simulink model "maze_solver"  (R2026a)
settings: Solver=FixedStepDiscrete  StopTime=1  FixedStep=0.01
InitFcn:
  | run(fullfile(currentProject().RootFolder,'config','robot_params.m'))
undefined symbols (not defined in the file): DiscIntNeverNeededParam, motor, robot, Ts
settings Model: Creator=richs  LastModifiedBy=richs

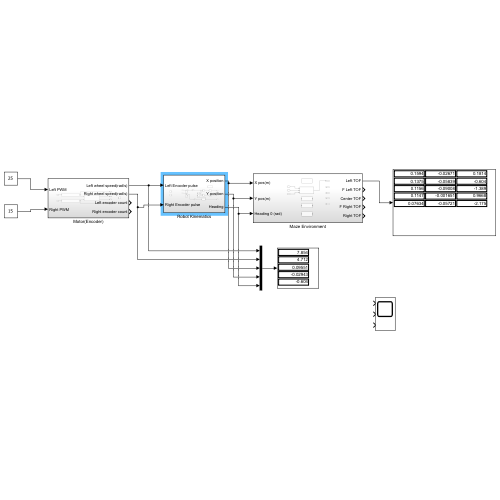
[thumbnail: Simulink's stored preview of the top-level diagram]
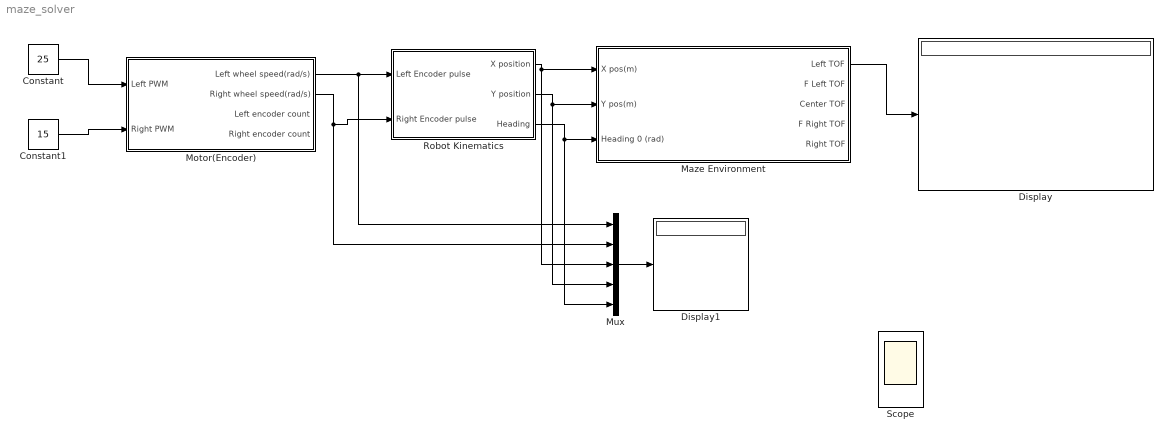
== system maze_solver ==
  Constant : Constant  Value=25
  Constant1 : Constant  Value=15
  Display : Display
  Display1 : Display
  Maze Environment : Subsystem
  Motor(Encoder) : Subsystem
  Mux : Mux  Inputs=5
  Robot Kinematics : Subsystem
  Scope : Scope  NumInputPorts=3
      settings: ActiveDisplayYMinimum=-0.29962469310207057  ActiveDisplayYMaximum=0.042415818455105447
  wires:
  Motor(Encoder)/1(Left wheel speed(rad/s)) -> Mux/1, Robot Kinematics/1(Left Encoder pulse)
  Motor(Encoder)/2(Right wheel speed(rad/s)) -> Mux/2, Robot Kinematics/2(Right Encoder pulse)
  Constant/1 -> Motor(Encoder)/1(Left PWM)
  Constant1/1 -> Motor(Encoder)/2(Right PWM)
  Robot Kinematics/1(X position) -> Mux/3, Maze Environment/1(X pos(m))
  Robot Kinematics/2(Y position) -> Mux/4, Maze Environment/2(Y pos(m))
  Robot Kinematics/3(Heading) -> Mux/5, Maze Environment/3(Heading 0 (rad))
  Mux/1 -> Display1/1
  Maze Environment/1(Left TOF) -> Display/1

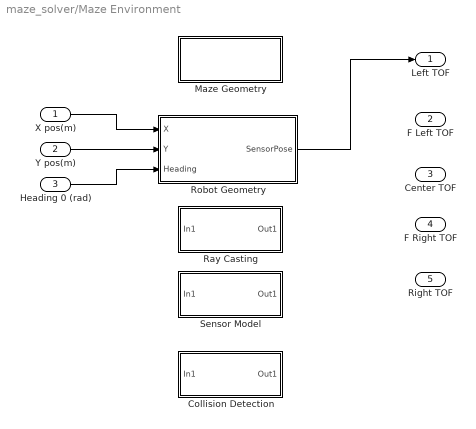
== system maze_solver/Maze Environment ==
  X pos(m) : Inport
  Y pos(m) : Inport  Port=2
  Heading 0 (rad) : Inport  Port=3
  Collision Detection : Subsystem
  Maze Geometry : Subsystem
  Ray Casting : Subsystem
  Robot Geometry : Subsystem
  Sensor Model : Subsystem
  Left TOF : Outport
  F Left TOF : Outport  Port=2
  Center TOF : Outport  Port=3
  F Right TOF : Outport  Port=4
  Right TOF : Outport  Port=5
  wires:
  X pos(m)/1 -> Robot Geometry/1(X)
  Y pos(m)/1 -> Robot Geometry/2(Y)
  Heading 0 (rad)/1 -> Robot Geometry/3(Heading)
  Robot Geometry/1(SensorPose) -> Left TOF/1

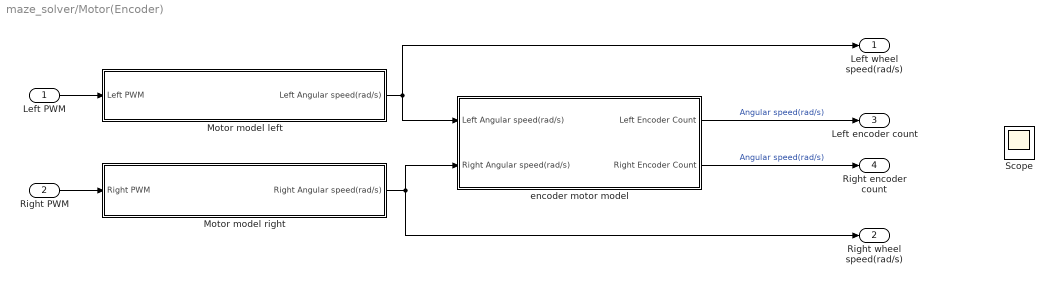
== system maze_solver/Motor(Encoder) ==
  Left PWM : Inport
  Right PWM : Inport  Port=2
  Motor model left : Subsystem
  Motor model right : Subsystem
  Scope : Scope  NumInputPorts=2
      settings: ActiveDisplayYMinimum=259.90483016263516  ActiveDisplayYMaximum=297.8633074912612
  encoder motor model : Subsystem
  Left wheel speed(rad/s) : Outport
  Right wheel speed(rad/s) : Outport  Port=2
  Left encoder count : Outport  Port=3
  Right encoder count : Outport  Port=4
  wires:
  Motor model left/1(Left Angular speed(rad/s)) -> encoder motor model/1(Left Angular speed(rad/s)), Left wheel speed(rad/s)/1
  Motor model right/1(Right Angular speed(rad/s)) -> Right wheel speed(rad/s)/1, encoder motor model/2(Right Angular speed(rad/s))
  Left PWM/1 -> Motor model left/1(Left PWM)
  Right PWM/1 -> Motor model right/1(Right PWM)
  encoder motor model/1(Left Encoder Count) -> Left encoder count/1  "Angular speed(rad/s)"
  encoder motor model/2(Right Encoder Count) -> Right encoder count/1  "Angular speed(rad/s)"

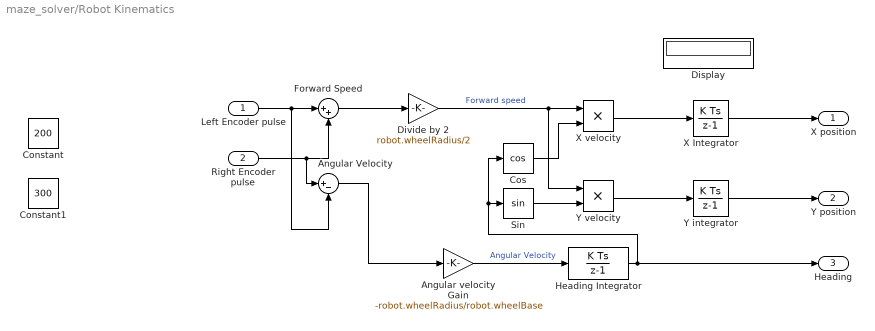
== system maze_solver/Robot Kinematics ==
  Left Encoder pulse : Inport
  Right Encoder pulse : Inport  Port=2
  " X velocity" : Product
  Angular Velocity : Sum  Inputs=|+-
  Angular velocity Gain : Gain  Gain=-robot.wheelRadius/robot.wheelBase
  Constant : Constant  Value=200
  Constant1 : Constant  Value=300
  Cos : Trigonometry  Operator=cos
  Display : Display
  Divide by 2 : Gain  Gain=robot.wheelRadius/2
  Forward Speed : Sum  Inputs=|++
  Heading Integrator : DiscreteIntegrator  SampleTime=Ts  ICPrevOutput=DiscIntNeverNeededParam  ICPrevScaledInput=DiscIntNeverNeededParam
  Sin : Trigonometry
  X Integrator : DiscreteIntegrator  SampleTime=Ts  ICPrevOutput=DiscIntNeverNeededParam  ICPrevScaledInput=DiscIntNeverNeededParam
  Y integrator : DiscreteIntegrator  SampleTime=Ts  ICPrevOutput=DiscIntNeverNeededParam  ICPrevScaledInput=DiscIntNeverNeededParam
  Y velocity : Product
  X position : Outport
  Y position : Outport  Port=2
  Heading : Outport  Port=3
  wires:
  Forward Speed/1 -> Divide by 2/1
  Divide by 2/1 -> Y velocity/1, " X velocity"/1  "Forward speed"
  Angular velocity Gain/1 -> Heading Integrator/1  "Angular Velocity"
  Cos/1 -> " X velocity"/2
  Sin/1 -> Y velocity/2
  " X velocity"/1 -> X Integrator/1
  Y velocity/1 -> Y integrator/1
  Y integrator/1 -> Y position/1
  X Integrator/1 -> X position/1
  Angular Velocity/1 -> Angular velocity Gain/1
  Heading Integrator/1 -> Heading/1, Cos/1, Sin/1
  Left Encoder pulse/1 -> Angular Velocity/2, Forward Speed/1
  Right Encoder pulse/1 -> Forward Speed/2, Angular Velocity/1

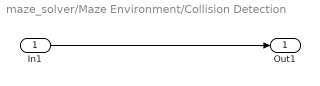
== system maze_solver/Maze Environment/Collision Detection ==
  In1 : Inport
  Out1 : Outport
  wires:
  In1/1 -> Out1/1

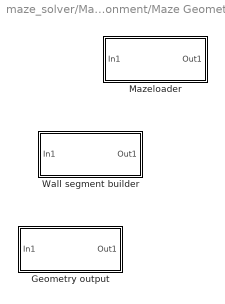
== system maze_solver/Maze Environment/Maze Geometry ==
  Geometry output : Subsystem
  Mazeloader : Subsystem
  Wall segment builder : Subsystem

== system maze_solver/Maze Environment/Ray Casting ==
  In1 : Inport
  Out1 : Outport
  wires:
  In1/1 -> Out1/1

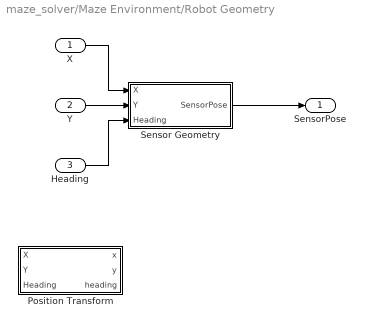
== system maze_solver/Maze Environment/Robot Geometry ==
  X : Inport
  Y : Inport  Port=2
  Heading : Inport  Port=3
  Position Transform : Subsystem
  Sensor Geometry : Subsystem
  SensorPose : Outport
  wires:
  Sensor Geometry/1(SensorPose) -> SensorPose/1
  X/1 -> Sensor Geometry/1(X)
  Y/1 -> Sensor Geometry/2(Y)
  Heading/1 -> Sensor Geometry/3(Heading)

== system maze_solver/Maze Environment/Sensor Model ==
  In1 : Inport
  Out1 : Outport
  wires:
  In1/1 -> Out1/1

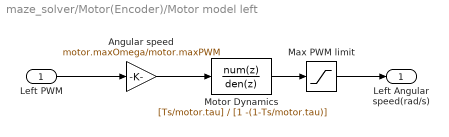
== system maze_solver/Motor(Encoder)/Motor model left ==
  Left PWM : Inport
  Angular speed : Gain  Gain=motor.maxOmega/motor.maxPWM
  Max PWM limit : Saturate  UpperLimit=motor.maxRPM  LowerLimit=-motor.maxRPM
  Motor Dynamics : DiscreteTransferFcn  Numerator=[Ts/motor.tau]  Denominator=[1 -(1-Ts/motor.tau)]
  Left Angular speed(rad/s) : Outport
  wires:
  Motor Dynamics/1 -> Max PWM limit/1
  Angular speed/1 -> Motor Dynamics/1
  Left PWM/1 -> Angular speed/1
  Max PWM limit/1 -> Left Angular speed(rad/s)/1

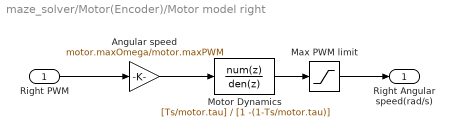
== system maze_solver/Motor(Encoder)/Motor model right ==
  Right PWM : Inport
  Angular speed : Gain  Gain=motor.maxOmega/motor.maxPWM
  Max PWM limit : Saturate  UpperLimit=motor.maxRPM  LowerLimit=-motor.maxRPM
  Motor Dynamics : DiscreteTransferFcn  Numerator=[Ts/motor.tau]  Denominator=[1 -(1-Ts/motor.tau)]
  Right Angular speed(rad/s) : Outport
  wires:
  Motor Dynamics/1 -> Max PWM limit/1
  Angular speed/1 -> Motor Dynamics/1
  Right PWM/1 -> Angular speed/1
  Max PWM limit/1 -> Right Angular speed(rad/s)/1

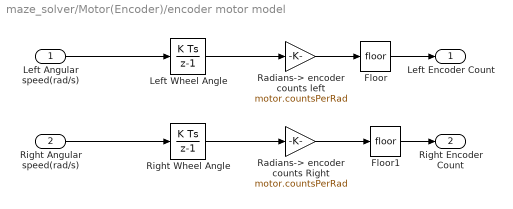
== system maze_solver/Motor(Encoder)/encoder motor model ==
  Left Angular speed(rad/s) : Inport
  Right Angular speed(rad/s) : Inport  Port=2
  Floor : Rounding
  Floor1 : Rounding
  Left Wheel Angle : DiscreteIntegrator  SampleTime=Ts  ICPrevOutput=DiscIntNeverNeededParam  ICPrevScaledInput=DiscIntNeverNeededParam
  Radians-> encoder counts left : Gain  Gain=motor.countsPerRad
  Radians-> encoder counts Right : Gain  Gain=motor.countsPerRad
  Right Wheel Angle : DiscreteIntegrator  SampleTime=Ts  ICPrevOutput=DiscIntNeverNeededParam  ICPrevScaledInput=DiscIntNeverNeededParam
  Left Encoder Count : Outport
  Right Encoder Count : Outport  Port=2
  wires:
  Left Angular speed(rad/s)/1 -> Left Wheel Angle/1
  Left Wheel Angle/1 -> Radians-> encoder counts left/1
  Radians-> encoder counts left/1 -> Floor/1
  Right Angular speed(rad/s)/1 -> Right Wheel Angle/1
  Right Wheel Angle/1 -> Radians-> encoder counts Right/1
  Radians-> encoder counts Right/1 -> Floor1/1
  Floor/1 -> Left Encoder Count/1
  Floor1/1 -> Right Encoder Count/1

== system maze_solver/Maze Environment/Maze Geometry/Geometry output ==
  In1 : Inport
  Out1 : Outport
  wires:
  In1/1 -> Out1/1

== system maze_solver/Maze Environment/Maze Geometry/Mazeloader ==
  In1 : Inport
  Out1 : Outport
  wires:
  In1/1 -> Out1/1

== system maze_solver/Maze Environment/Maze Geometry/Wall segment builder ==
  In1 : Inport
  Out1 : Outport
  wires:
  In1/1 -> Out1/1

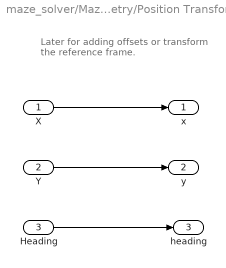
== system maze_solver/Maze Environment/Robot Geometry/Position Transform ==
  note: Later for adding offsets or transform
      | the reference frame.
  X : Inport
  Y : Inport  Port=2
  Heading : Inport  Port=3
  x : Outport
  y : Outport  Port=2
  heading : Outport  Port=3
  wires:
  X/1 -> x/1
  Y/1 -> y/1
  Heading/1 -> heading/1

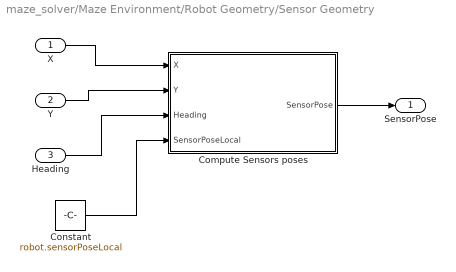
== system maze_solver/Maze Environment/Robot Geometry/Sensor Geometry ==
  X : Inport
  Y : Inport  Port=2
  Heading : Inport  Port=3
  Compute Sensors poses : MATLAB Function  TreatAsAtomicUnit=on
  Constant : Constant  Value=robot.sensorPoseLocal
  SensorPose : Outport
  wires:
  X/1 -> Compute Sensors poses/1(X)
  Y/1 -> Compute Sensors poses/2(Y)
  Heading/1 -> Compute Sensors poses/3(Heading)
  Compute Sensors poses/1(SensorPose) -> SensorPose/1
  Constant/1 -> Compute Sensors poses/4(SensorPoseLocal)

== matlab function maze_solver/Maze Environment/Robot Geometry/Sensor Geometry/Compute Sensors poses ==
  data: X input; SensorPose output; Y input; Heading input; SensorPoseLocal input
function SensorPose = ComputeSensorPoses(X,Y,Heading,SensorPoseLocal)

% Allocate output
SensorPose = zeros(5,3);

% Rotation terms
c = cos(Heading);
s = sin(Heading);

% Compute world pose of each sensor
for i = 1:5

    xLocal = SensorPoseLocal(i,1);
    yLocal = SensorPoseLocal(i,2);
    thetaLocal = SensorPoseLocal(i,3);

    xWorld = X + xLocal*c - yLocal*s;
    yWorld = Y + xLocal*s + yLocal*c;
    thetaWorld = Heading + thetaLocal;

    SensorPose(i,:) = [xWorld yWorld thetaWorld];

end

end
